simulink model "Field_Oriented_Control_of_IM"  (R2019a)
settings: Solver=VariableStepAuto  StartTime=0.0  StopTime=13  RelTol=1e-3
undefined symbols (not defined in the file): DiscIntNeverNeededParam
libraries: powerlib x4, simulink x2, powerlib_meascontrol x2
settings Model: Creator=Deepak  LastModifiedBy=Deepak

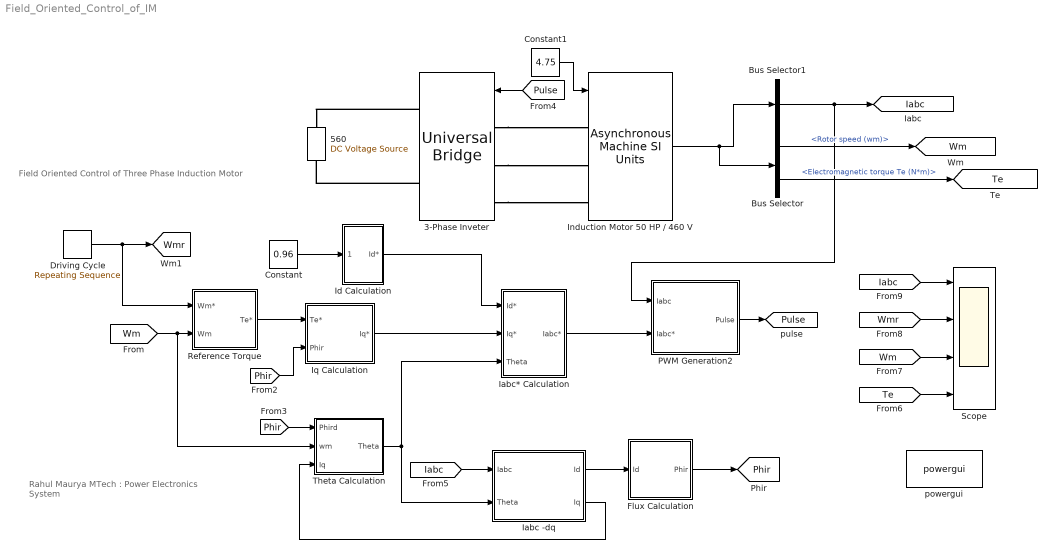
== system Field_Oriented_Control_of_IM ==
  note: Rahul Maurya
      | MTech : Power Electronics System
  note: Field Oriented Control of Three Phase Induction Motor
  3-Phase Inveter : powerlib/Power Electronics/Universal Bridge  Arms=3  SnubberResistance=1e5  SnubberCapacitance=1e-6  Device=IGBT / Diodes  Ron=1e-3  Lon=0  ForwardVoltages="[1.1  0.75]"  ForwardVoltage=0  GTOparameters=[ 10e-6 , 20e-6 ]  IGBTparameters=[ 1e-6 , 2e-6 ]  Measurements=None  Measurements_2=None  converterType=Rectifier
      settings: SourceProductName=Simscape Electrical
  560 : powerlib/Electrical Sources/DC Voltage Source  Amplitude=530  Measurements=None
      settings: SourceProductName=Simscape Electrical
  Bus Selector : BusSelector  OutputSignals=Mechanical.Rotor speed (wm),Mechanical.Electromagnetic torque Te (N*m)
  Bus Selector1 : BusSelector  OutputSignals=Stator measurements.Stator current is_a (A),Stator measurements.Stator current is_b (A),Stator measurements.Stator current is_c (A)  OutputAsBus=on
  Constant : Constant  Value=0.96
  Constant1 : Constant  Value=4.75
  Driving Cycle : simulink/Sources/Repeating Sequence  rep_seq_t=[0 1 2 3 4 5 6 7 8 9 10 11 11.0001 12 13]  rep_seq_y=[0 0 20 20 0 0 30 30 0 0 50 50 40 40 0]
  Flux Calculation : Subsystem
  Iabc -dq : Subsystem
  "Iabc* Calculation " : Subsystem
  Id Calculation : Subsystem
  Induction Motor 50 HP / 460 V : powerlib/Machines/Asynchronous Machine SI Units  RotorType=Squirrel-cage  PresetModel=No  MechanicalLoad=Torque Tm  ShowDetailedParameters=on  ReferenceFrame=Stationary  Units=SI  MeasurementBus=off  NominalParameters=[ 50*746, 460, 60 ]  Stator=[ 0.087 0.8e-3 ]  Rotor="[ 0.228  0.8e-3 ]"  Cage1=[0.4155 0.002066]  Cage2=[0.4168 0.0003495]  Lm=34.7e-3  Mechanical="[1.662  0.01 2 ]"  PolePairs=2  InitialConditions="[ 1, 0 ,  0 , 0 , 0 , 0 , 0 , 0 ]"  SimulateSaturation=off  Saturation=[0 0;0 0]  LoadFlowParameters=0  TsPowergui=0  TsBlock=-1  IterativeModel=Trapezoidal non iterative  IterativeDiscreteModel=Trapezoidal non iterative  Pmec=1.492e+006
      settings: SourceProductName=Simscape Electrical
  Iq Calculation : Subsystem
  PWM Generation2 : Subsystem
  Reference Torque : Subsystem
  Scope : Scope  NumInputPorts=4
  Theta Calculation : Subsystem
  powergui : powerlib/powergui  Priority=1  SimulationMode=Discrete  SampleTime=2e-6  frequency=60  Iterations=50  frequencyindice=60  Pbase=100e6  ErrMax=1e-4  UnitsV=kV  UnitsW=MW  buscounter=0  FunctionMessages=off  echomessages=off  EnableUseOfTLC=off  CurrentSourceSwitches=off  DisableSnubberDevices=off  DisableRonSwitches=off  DisableVfSwitches=off  DisplayEquations=off  AutomaticDiscreteSolvers=off  SolverType=Tustin/Backward Euler (TBE)  Interpol=off  ExternalGateDelay=off  methode=off  Ts=100  x0status=blocks  SPID=on  SwTol=0  HookPort=off  NonlinearTolerance=0  nMaxIteration=15  ContinueOnMaxIteration=off  RestoreLinks=warning  ResistiveCurrentMeasurement=off  Frange=[0:2:500]  Ylog=off  Xlog=on  ShowGrid=off  save=off  variable=ZData  structure=0  ZoomFFT=off  StartTime=0.0  cycles=1  DisplayStyle=1  fundamental=60  FreqAxis=off  MaxFrequency=1000  frequencyindicesteady=1  RmsSteady=1  display=off
      settings: SourceProductName=Simscape Electrical
  tag scope: Iabc=global, Phir=global, Pulse=global, Te=global, Wm=global, Wmr=global
  wires:
  Induction Motor 50 HP / 460 V/1 -> Bus Selector/1, Bus Selector1/1
  Bus Selector/1 -> [Wm]  "<Rotor speed (wm)>"
  Bus Selector/2 -> [Te]  "<Electromagnetic torque Te (N*m)>"
  Reference Torque/1(Te*) -> Iq Calculation/1(Te*)
  Iq Calculation/1(Iq*) -> "Iabc* Calculation "/2(Iq*)
  Theta Calculation/1(Theta) -> "Iabc* Calculation "/3(Theta), Iabc -dq/2(Theta)
  Flux Calculation/1(Phir) -> [Phir]
  [Phir] -> Iq Calculation/2(Phir)
  [Iabc] -> Iabc -dq/1(Iabc)
  Id Calculation/1(Id*) -> "Iabc* Calculation "/1(Id*)
  Constant/1 -> Id Calculation/1(Phir*)
  [Pulse] -> 3-Phase Inveter/1
  [Wm] -> Scope/3
  [Te] -> Scope/4
  [Wmr] -> Scope/2
  [Iabc] -> Scope/1
  Constant1/1 -> Induction Motor 50 HP / 460 V/1
  Bus Selector1/1 -> PWM Generation2/1(Iabc), [Iabc]
  Iabc -dq/1(Id) -> Flux Calculation/1(Id)
  [Phir] -> Theta Calculation/1(Phird)
  [Wm] -> Theta Calculation/2(wm), Reference Torque/2(Wm)
  "Iabc* Calculation "/1(Iabc*) -> PWM Generation2/2(Iabc*)
  PWM Generation2/1(Pulse) -> [Pulse]
  Driving Cycle/1 -> Reference Torque/1(Wm*), [Wmr]
  Iabc -dq/2(Iq) -> Theta Calculation/3(Iq)
  connections:
  3-Phase Inveter/RConn2 -- 560/LConn1
  3-Phase Inveter/LConn1 -- Induction Motor 50 HP / 460 V/LConn1
  3-Phase Inveter/LConn2 -- Induction Motor 50 HP / 460 V/LConn2
  3-Phase Inveter/LConn3 -- Induction Motor 50 HP / 460 V/LConn3
  3-Phase Inveter/RConn1 -- 560/RConn1

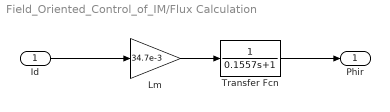
== system Field_Oriented_Control_of_IM/Flux Calculation ==
  Id : Inport
  Lm : Gain  Gain=34.7e-3
  Transfer Fcn : TransferFcn  Denominator=[0.1557 1]
  Phir : Outport
  wires:
  Id/1 -> Lm/1
  Lm/1 -> Transfer Fcn/1
  Transfer Fcn/1 -> Phir/1

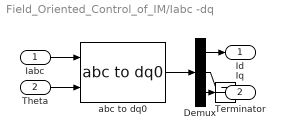
== system Field_Oriented_Control_of_IM/Iabc -dq ==
  Iabc : Inport
  Theta : Inport  Port=2
  Demux : Demux  Outputs=3
  Terminator : Terminator
  abc to dq0 : powerlib_meascontrol/Transformations/abc to dq0  Alignment=90 degrees behind phase A axis
      settings: SourceProductName=Simscape Electrical
  Id : Outport
  Iq : Outport  Port=2
  wires:
  Demux/3 -> Terminator/1
  abc to dq0/1 -> Demux/1
  Demux/2 -> Iq/1
  Theta/1 -> abc to dq0/2
  Iabc/1 -> abc to dq0/1
  Demux/1 -> Id/1

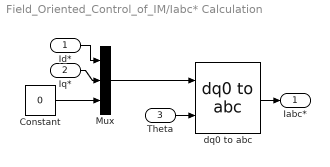
== system Field_Oriented_Control_of_IM/Iabc* Calculation  ==
  Id* : Inport
  Iq* : Inport  Port=2
  Theta : Inport  Port=3
  Constant : Constant  Value=0
  Mux : Mux  Inputs=3
  dq0 to abc : powerlib_meascontrol/Transformations/dq0 to abc  Alignment=90 degrees behind phase A axis
      settings: SourceProductName=Simscape Electrical
  Iabc* : Outport
  wires:
  dq0 to abc/1 -> Iabc*/1
  Id*/1 -> Mux/1
  Constant/1 -> Mux/3
  Iq*/1 -> Mux/2
  Mux/1 -> dq0 to abc/1
  Theta/1 -> dq0 to abc/2

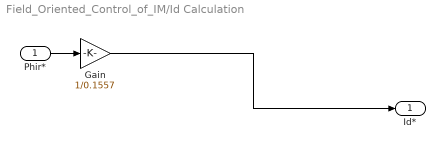
== system Field_Oriented_Control_of_IM/Id Calculation ==
  Phir* : Inport
  Gain : Gain  Gain=1/0.1557
  Id* : Outport
  wires:
  Phir*/1 -> Gain/1
  Gain/1 -> Id*/1

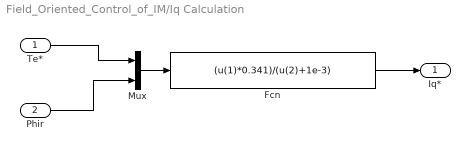
== system Field_Oriented_Control_of_IM/Iq Calculation ==
  Te* : Inport
  Phir : Inport  Port=2
  Fcn : Fcn  Expr=(u(1)*0.341)/(u(2)+1e-3)
  Mux : Mux  Inputs=2
  Iq* : Outport
  wires:
  Fcn/1 -> Iq*/1
  Mux/1 -> Fcn/1
  Phir/1 -> Mux/2
  Te*/1 -> Mux/1

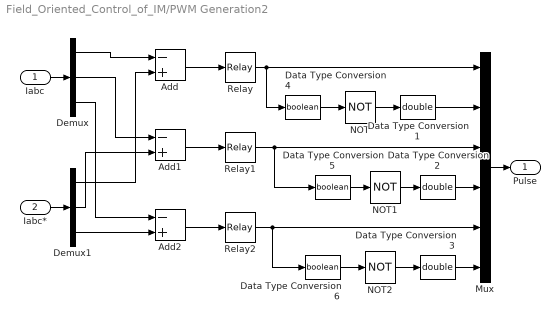
== system Field_Oriented_Control_of_IM/PWM Generation2 ==
  Iabc : Inport
  Iabc* : Inport  Port=2
  Add : Sum  Inputs=-+
  Add1 : Sum  Inputs=-+
  Add2 : Sum  Inputs=-+
  Data Type Conversion1 : DataTypeConversion  OutDataTypeStr=double
  Data Type Conversion2 : DataTypeConversion  OutDataTypeStr=double
  Data Type Conversion3 : DataTypeConversion  OutDataTypeStr=double
  Data Type Conversion4 : DataTypeConversion  OutDataTypeStr=boolean
  Data Type Conversion5 : DataTypeConversion  OutDataTypeStr=boolean
  Data Type Conversion6 : DataTypeConversion  OutDataTypeStr=boolean
  Demux : Demux  Outputs=3
  Demux1 : Demux  Outputs=3
  Mux : Mux  Inputs=6
  NOT : Logic  Operator=NOT  AllPortsSameDT=off  OutDataTypeStr=boolean
  NOT1 : Logic  Operator=NOT  AllPortsSameDT=off  OutDataTypeStr=boolean
  NOT2 : Logic  Operator=NOT  AllPortsSameDT=off  OutDataTypeStr=boolean
  Relay : Relay
  Relay1 : Relay
  Relay2 : Relay
  Pulse : Outport
  wires:
  Add/1 -> Relay/1
  Relay1/1 -> Data Type Conversion5/1, Mux/3
  NOT/1 -> Data Type Conversion1/1
  Demux1/1 -> Add/2
  Data Type Conversion4/1 -> NOT/1
  Data Type Conversion6/1 -> NOT2/1
  Relay2/1 -> Data Type Conversion6/1, Mux/5
  Mux/1 -> Pulse/1
  Relay/1 -> Data Type Conversion4/1, Mux/1
  Data Type Conversion1/1 -> Mux/2
  Data Type Conversion2/1 -> Mux/4
  Data Type Conversion3/1 -> Mux/6
  Add2/1 -> Relay2/1
  Iabc*/1 -> Demux1/1
  Add1/1 -> Relay1/1
  Data Type Conversion5/1 -> NOT1/1
  NOT2/1 -> Data Type Conversion3/1
  Demux1/2 -> Add1/2
  Demux/2 -> Add1/1
  Demux1/3 -> Add2/2
  Demux/1 -> Add/1
  NOT1/1 -> Data Type Conversion2/1
  Demux/3 -> Add2/1
  Iabc/1 -> Demux/1

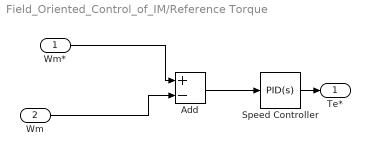
== system Field_Oriented_Control_of_IM/Reference Torque ==
  Wm* : Inport
  Wm : Inport  Port=2
  Add : Sum  Inputs=+-
  Speed Controller : simulink/Continuous/PID Controller  Controller=PID  Form=Parallel  TimeDomain=Continuous-time  SampleTime=2e-6  IntegratorMethod=Forward Euler  FilterMethod=Forward Euler  ControllerParametersSource=internal  P=13  I=26  D=0  UseFilter=on  N=100  TunerSelectOption=Transfer Function Based (PID Tuner App)  InitialConditionSource=internal  InitialConditionForIntegrator=50  InitialConditionForFilter=0  DifferentiatorICPrevScaledInput=0  ExternalReset=none  TrackingMode=off  Kt=1  LimitOutput=on  UpperSaturationLimit=200  LowerSaturationLimit=-200  LinearizeAsGain=off  AntiWindupMode=clamping  Kb=1  POutMin=[]  POutMax=[]  IOutMin=[]  IOutMax=[]  DOutMin=[]  DOutMax=[]  NOutMin=[]  NOutMax=[]  SumOutMin=[]  SumOutMax=[]  SaturationOutMin=[]  SaturationOutMax=[]  PParamMin=[]  PParamMax=[]  IParamMin=[]  IParamMax=[]  DParamMin=[]  DParamMax=[]  NParamMin=[]  NParamMax=[]  KbParamMin=[]  KbParamMax=[]  KtParamMin=[]  KtParamMax=[]  KbOutMin=[]  KbOutMax=[]  KtOutMin=[]  KtOutMax=[]  IntegratorOutMin=[]  IntegratorOutMax=[]  FilterOutMin=[]  FilterOutMax=[]  SumI1OutMin=[]  SumI1OutMax=[]  SumI2OutMin=[]  SumI2OutMax=[]  SumI3OutMin=[]  SumI3OutMax=[]  SumI4OutMin=[]  SumI4OutMax=[]  SumDOutMin=[]  SumDOutMax=[]  DifferentiatorOutMin=[]  DifferentiatorOutMax=[]  FilterDiffOutCoefMin=[]  FilterDiffOutCoefMax=[]  ReciprocalOutMin=[]  ReciprocalOutMax=[]  SumDenOutMin=[]  SumDenOutMax=[]  SumNumOutMin=[]  SumNumOutMax=[]  DivideOutMin=[]  DivideOutMax=[]  IntegratorContinuousStateAttributes=''  IntegratorStateMustResolveToSignalObject=off  IntegratorRTWStateStorageClass=Auto  FilterContinuousStateAttributes=''  FilterStateMustResolveToSignalObject=off  FilterRTWStateStorageClass=Auto  ParallelPVariant=InternalParameters  IdealPVariant=Disabled  IVariant=InternalParameters  DVariant=InternalParameters  IntegratorVariant=Continuous  SatVariant=Enabled  AWVariant=ContClampingParallel  PCopyVariant=Disabled  TRVariant=Disabled  FdbkBlocksVariant=Forward  IdealPFdbkVariant=Disabled  SatFdbkVariant=Disabled  DerivativeFilterVariant=ContFilter  NVariant=InternalParameters  NCopyVariant=Disabled  FilterICVariant=InternalICsFilter  IntegratorICVariant=InternalICs  ExternalResetVariant=Disabled  TRSumVariant=Passthrough  SumFdbkVariant=Disabled  SumVariant=Sum_PID
  Te* : Outport
  wires:
  Add/1 -> Speed Controller/1
  Speed Controller/1 -> Te*/1
  Wm/1 -> Add/2
  Wm*/1 -> Add/1

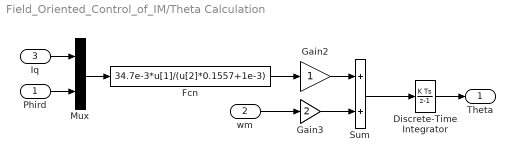
== system Field_Oriented_Control_of_IM/Theta Calculation ==
  Phird : Inport
  wm : Inport  Port=2
  Iq : Inport  Port=3
  Discrete-Time Integrator : DiscreteIntegrator  SampleTime=1e-5  ICPrevOutput=DiscIntNeverNeededParam  ICPrevScaledInput=DiscIntNeverNeededParam
  Fcn : Fcn  Expr=34.7e-3*u[1]/(u[2]*0.1557+1e-3)
  Gain2 : Gain  SaturateOnIntegerOverflow=on  OutDataTypeStr=Inherit: Same as input  ParamDataTypeStr=Inherit: Same as input
  Gain3 : Gain  Gain=2  SaturateOnIntegerOverflow=on  OutDataTypeStr=Inherit: Same as input  ParamDataTypeStr=Inherit: Same as input
  Mux : Mux  Inputs=2
  Sum : Sum  SaturateOnIntegerOverflow=on  InputSameDT=on  OutDataTypeStr=Inherit: Same as first input
  Theta : Outport  InitialOutput=0
  wires:
  Fcn/1 -> Gain2/1
  Mux/1 -> Fcn/1
  Iq/1 -> Mux/1
  Gain3/1 -> Sum/2
  wm/1 -> Gain3/1
  Sum/1 -> Discrete-Time Integrator/1
  Phird/1 -> Mux/2
  Discrete-Time Integrator/1 -> Theta/1
  Gain2/1 -> Sum/1
